simulink model "FPIDUpravlenie"  (Simulink 7.7)
settings: Solver=ode23t  StartTime=0.0  StopTime=50  RelTol=1e-3
values from neighbouring files (symbols this model uses):
  control_a = [-1,-0.975000000000000,-0.950000000000000,-0.925000000000000,-0.900000000000000,-0.875000000000000,-0.850000000000000,-0.825000000000000,-0.800000000000000,-0.775000000000000,-0.750000000000000,-0.725000000000000,-0.700000000000000,-0.675000000000000,-0.650000000000000,-0.625000000000000,-0.600000000000000,-0.575000000000000,-0.550000000000000,-0.525000000000000,-0.500000000000000,-0.4750000000000 ...(+1058 chars)    [main.m]
  control_p = [-1,-0.975000000000000,-0.950000000000000,-0.925000000000000,-0.900000000000000,-0.875000000000000,-0.850000000000000,-0.825000000000000,-0.800000000000000,-0.775000000000000,-0.750000000000000,-0.725000000000000,-0.700000000000000,-0.675000000000000,-0.650000000000000,-0.625000000000000,-0.600000000000000,-0.575000000000000,-0.550000000000000,-0.525000000000000,-0.500000000000000,-0.4750000000000 ...(+1058 chars)    [main.m]
  force_a = [-1.11662323915155,-1.09378407342940,-1.07265330175950,-1.04325193963191,-1.01132720072323,-0.977223749190414,-0.938313974120250,-0.915271484375000,-0.878089162348878,-0.843089432210708,-0.808883264518567,-0.764209831066494,-0.722158864286485,-0.679419665506261,-0.643924317249568,-0.610622608349525,-0.566994046173359,-0.526776706201425,-0.495851299384715,-0.457681114394430,-0.413805712974957,-0.38 ...(+1125 chars)    [main.m]
  force_p = [-0.714170782059585,-0.698541481136658,-0.676359428972366,-0.657306593399180,-0.636149510200777,-0.615949677515112,-0.602138570676813,-0.585879142379102,-0.565408182885363,-0.543655801354706,-0.527755120628238,-0.502405059234672,-0.485276085519214,-0.468134124703152,-0.445933772533463,-0.427151136118307,-0.408462867012090,-0.386931266191710,-0.367853637062824,-0.349068470693005,-0.324248856460492, ...(+1121 chars)    [main.m]
  Kpa = 0.7*Kua    (= 0.465009225034)    [main.m]
  Kpp = 0.33*Kup    (= 0.127856690685)    [main.m]
  rpm_a = [-7339.45782001209,-7212.46690016528,-7085.45931302586,-6928.76328688402,-6788.57281024633,-6657.59465144230,-6511.41380896936,-6365.92031625604,-6207.93597881609,-6041.64663461541,-5911.49080716649,-5761.94058931792,-5622.99053485574,-5477.24984975964,-5308.98813100961,-5148.14194899341,-4993.59811636119,-4838.25096717246,-4657.71766075724,-4490.92806302583,-4332.56953312800,-4153.59004094051,-39 ...(+1020 chars)    [main.m]
  rpm_p = [-3941.33990805745,-3812.34781047405,-3751.11151919774,-3716.53325007516,-3652.15015900441,-3605.21060614596,-3541.61821912219,-3501.87845652477,-3434.16395565290,-3361.65746230900,-3323.64747018525,-3262.37352633531,-3200.40694372361,-3113.97714681560,-3066.79116629220,-2985.72573717380,-2938.26747796475,-2854.00073711688,-2797.89727840112,-2739.44446768238,-2641.03778047718,-2564.22034843818,-24 ...(+1020 chars)    [main.m]
  Tda = 0.15*Tua    (= 1.125)    [main.m]
  Tdp = 0.33*Tup    (= 0.825)    [main.m]
  Tia = 0.4*Tua    (= 3)    [main.m]
  Tip = 0.5*Tup    (= 1.25)    [main.m]
  Ts = 0.1    [main.m]
undefined symbols (not defined in the file or in its folder): DiscIntNeverNeededParam
libraries: simulink x6, fuzblock x2
settings Model: Creator=melanholly  LastModifiedBy=melanholly
settings SolverCC: ShapePreserveControl=EnableAll  SolverResetMethod=Robust

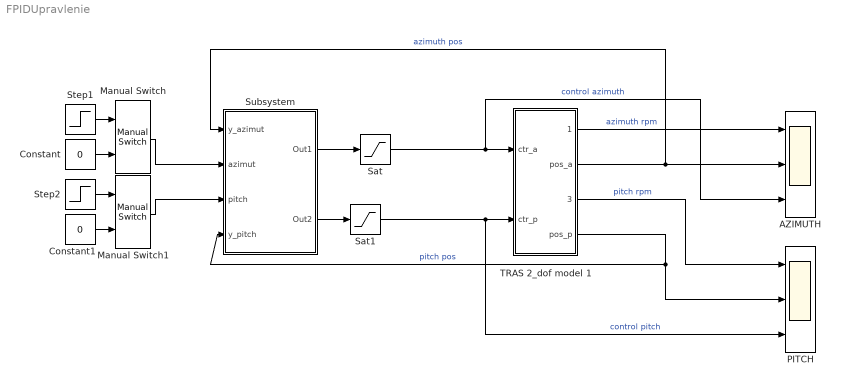
== system FPIDUpravlenie ==
  AZIMUTH : Scope  NumInputPorts=3
      settings: TimeRange=50  YMin=-3000~0~-0.4  YMax=3000~1.5~0.4
  Constant : Constant  Value=0
  Constant1 : Constant  Value=0
  Manual Switch : simulink/Signal Routing/Manual Switch  SystemSampleTime=-1  sw=1  action=0  varsize=off
  Manual Switch1 : simulink/Signal Routing/Manual Switch  SystemSampleTime=-1  sw=1  action=0  varsize=off
  PITCH : Scope  NumInputPorts=3
      settings: TimeRange=50  YMin=0~-2~0.2  YMax=4000~2~1
  Sat : Saturate  UpperLimit=0.3  LowerLimit=-0.3
  Sat1 : Saturate  UpperLimit=1  LowerLimit=.2
  Step1 : Step  After=0.3  SampleTime=0
  Step2 : Step  After=0.3  SampleTime=0
  Subsystem : Subsystem  mask{Kp_a=Kpa, Ki_a=Kpa/Tia, Kd_a=Kpa*Tda, Kp2=0, Ti2=0, Td2=0.2, N2=1, Kp3=0, Ti3=0, Td3=0.2, N3=1, Kp_p=Kpp, Ki_p=Kpp/Tip, Kd_p=Kpp*Tdp}
      mask prompts: Kp_a "Kp"; Ki_a "Ki"; Kd_a "Kd"; Kp2 "Kp"; Ti2 "Ti"; Td2 "Td"; N2 "N"; Kp3 "Kp"; Ti3 "Ti"; Td3 "Td"; N3 "N"; Kp_p "Kp"; Ki_p "Ki"; Kd_p "Kd"
      mask init:
      | GE_a = 1;
      | GCE_a = GE_a*(Kp_a-sqrt(Kp_a^2-4*Ki_a*Kd_a))/2/Ki_a;
      | GCU_a = Ki_a/GE_a;
      | GU_a = Kd_a/GCE_a;
      | if imag(GCE_a)~=0
      | error('GCE_a e kompleksno chislo molq promenenete koeficientite za nego');
      | end
      | 
      | GE_p = 1;
      | GCE_p = GE_p*(Kp_p-sqrt(Kp_p^2-4*Ki_p*Kd_p))/2/Ki_p;
      | GCU_p = Ki_p/GE_p;
      | GU_p = Kd_p/GCE_p;
      | 
      | if imag(GCE_p)~=0
      | error('GCE_p e kompleksno chislo molq promenenete koeficientite za nego');
      | end
      mask TabNameString: Azimut,Azimut,Azimut,hv,hv,hv,hv,vh,vh,vh,vh,Pitch,Pitch,Pitch
      mask Display:
      | disp Control
      | port_label('input', 1, 'a_y');
      | port_label('input', 2, 'a_r');
      | port_label('input', 3, 'p_r');
      | port_label('input', 4, 'p_y');
      | port_label('output', 1, 'ac');
      | port_label('output', 2, 'pc');
  TRAS 2_dof model 1 : Subsystem
  wires:
  TRAS 2_dof model 1/1(rpm_a) -> AZIMUTH/1  "azimuth rpm"
  TRAS 2_dof model 1/2(pos_a) -> AZIMUTH/2, Subsystem/1(y_azimut)  "azimuth pos"
  Step1/1 -> Manual Switch/1
  Constant/1 -> Manual Switch/2
  Step2/1 -> Manual Switch1/1
  Constant1/1 -> Manual Switch1/2
  TRAS 2_dof model 1/3(rpm_p) -> PITCH/1  "pitch rpm"
  TRAS 2_dof model 1/4(pos_p) -> PITCH/2, Subsystem/4(y_pitch)  "pitch pos"
  Manual Switch1/1 -> Subsystem/3(pitch)
  Subsystem/1(Out1) -> Sat/1
  Manual Switch/1 -> Subsystem/2(azimut)
  Sat1/1 -> PITCH/3, TRAS 2_dof model 1/2(ctr_p)  "control pitch"
  Sat/1 -> AZIMUTH/3, TRAS 2_dof model 1/1(ctr_a)  "control azimuth"
  Subsystem/2(Out2) -> Sat1/1

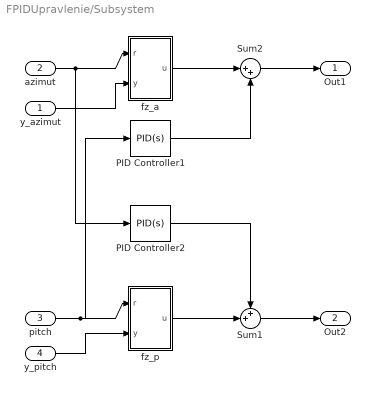
== system FPIDUpravlenie/Subsystem ==
  y_azimut : Inport
  azimut : Inport  Port=2
  pitch : Inport  Port=3
  y_pitch : Inport  Port=4
  PID Controller1 : simulink/Continuous/PID Controller  SystemSampleTime=-1  Controller=PID  TimeDomain=Continuous-time  SampleTime=1  IntegratorMethod=Forward Euler  FilterMethod=Forward Euler  Form=Ideal  P=Kp2  I=Ti2  D=Td2  N=N2  InitialConditionSource=internal  InitialConditionForIntegrator=0  InitialConditionForFilter=0  ExternalReset=none  LimitOutput=off  UpperSaturationLimit=inf  LowerSaturationLimit=-inf  LinearizeAsGain=off  AntiWindupMode=none  Kb=1  TrackingMode=off  Kt=1  PParamMin=[]  PParamMax=[]  IParamMin=[]  IParamMax=[]  DParamMin=[]  DParamMax=[]  NParamMin=[]  NParamMax=[]  KbParamMin=[]  KbParamMax=[]  KtParamMin=[]  KtParamMax=[]  POutMin=[]  POutMax=[]  IOutMin=[]  IOutMax=[]  DOutMin=[]  DOutMax=[]  NOutMin=[]  NOutMax=[]  KbOutMin=[]  KbOutMax=[]  KtOutMin=[]  KtOutMax=[]  IntegratorOutMin=[]  IntegratorOutMax=[]  FilterOutMin=[]  FilterOutMax=[]  SumOutMin=[]  SumOutMax=[]  SumI1OutMin=[]  SumI1OutMax=[]  SumI2OutMin=[]  SumI2OutMax=[]  SumI3OutMin=[]  SumI3OutMax=[]  SumDOutMin=[]  SumDOutMax=[]  SaturationOutMin=[]  SaturationOutMax=[]  IntegratorContinuousStateAttributes=''  IntegratorStateMustResolveToSignalObject=off  IntegratorRTWStateStorageClass=Auto  FilterContinuousStateAttributes=''  FilterStateMustResolveToSignalObject=off  FilterRTWStateStorageClass=Auto
  PID Controller2 : simulink/Continuous/PID Controller  SystemSampleTime=-1  Controller=PID  TimeDomain=Continuous-time  SampleTime=1  IntegratorMethod=Forward Euler  FilterMethod=Forward Euler  Form=Ideal  P=Kp3  I=Ti3  D=Td3  N=N3  InitialConditionSource=internal  InitialConditionForIntegrator=0  InitialConditionForFilter=0  ExternalReset=none  LimitOutput=off  UpperSaturationLimit=inf  LowerSaturationLimit=-inf  LinearizeAsGain=off  AntiWindupMode=none  Kb=1  TrackingMode=off  Kt=1  PParamMin=[]  PParamMax=[]  IParamMin=[]  IParamMax=[]  DParamMin=[]  DParamMax=[]  NParamMin=[]  NParamMax=[]  KbParamMin=[]  KbParamMax=[]  KtParamMin=[]  KtParamMax=[]  POutMin=[]  POutMax=[]  IOutMin=[]  IOutMax=[]  DOutMin=[]  DOutMax=[]  NOutMin=[]  NOutMax=[]  KbOutMin=[]  KbOutMax=[]  KtOutMin=[]  KtOutMax=[]  IntegratorOutMin=[]  IntegratorOutMax=[]  FilterOutMin=[]  FilterOutMax=[]  SumOutMin=[]  SumOutMax=[]  SumI1OutMin=[]  SumI1OutMax=[]  SumI2OutMin=[]  SumI2OutMax=[]  SumI3OutMin=[]  SumI3OutMax=[]  SumDOutMin=[]  SumDOutMax=[]  SaturationOutMin=[]  SaturationOutMax=[]  IntegratorContinuousStateAttributes=''  IntegratorStateMustResolveToSignalObject=off  IntegratorRTWStateStorageClass=Auto  FilterContinuousStateAttributes=''  FilterStateMustResolveToSignalObject=off  FilterRTWStateStorageClass=Auto
  Sum1 : Sum  Inputs=++|
  Sum2 : Sum  Inputs=|++
  fz_a : Subsystem
  fz_p : Subsystem
  Out1 : Outport
  Out2 : Outport  Port=2
  wires:
  azimut/1 -> PID Controller2/1, fz_a/1(r)
  pitch/1 -> PID Controller1/1, fz_p/1(r)
  PID Controller2/1 -> Sum1/1
  fz_p/1(u) -> Sum1/2
  Sum1/1 -> Out2/1
  fz_a/1(u) -> Sum2/1
  Sum2/1 -> Out1/1
  PID Controller1/1 -> Sum2/2
  y_azimut/1 -> fz_a/2(y)
  y_pitch/1 -> fz_p/2(y)

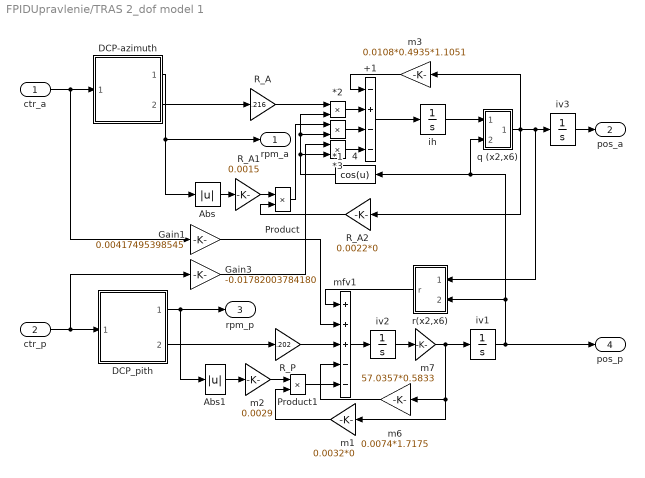
== system FPIDUpravlenie/TRAS 2_dof model 1 ==
  ctr_a : Inport
  ctr_p : Inport  Port=2
  *1 : Product  SaturateOnIntegerOverflow=on  InputSameDT=on  OutDataTypeStr=Inherit: Same as first input
  *2 : Product  SaturateOnIntegerOverflow=on  InputSameDT=on  OutDataTypeStr=Inherit: Same as first input
  *3 : Product  SaturateOnIntegerOverflow=on  InputSameDT=on  OutDataTypeStr=Inherit: Same as first input
  +1 : Sum  Inputs=-+--  SaturateOnIntegerOverflow=on  InputSameDT=on  OutDataTypeStr=Inherit: Same as first input
  4 : Fcn  Expr=cos(u)
  Abs : Abs  SaturateOnIntegerOverflow=on
  Abs1 : Abs  SaturateOnIntegerOverflow=on
  DCP-azimuth : Subsystem
  DCP_pith : Subsystem
  Gain1 : Gain  Gain=0.00417495398545  SaturateOnIntegerOverflow=on  OutDataTypeStr=Inherit: Same as input  ParamDataTypeStr=Inherit: Same as input
  Gain3 : Gain  Gain=-0.01782003784180  SaturateOnIntegerOverflow=on  OutDataTypeStr=Inherit: Same as input  ParamDataTypeStr=Inherit: Same as input
  Product : Product  SaturateOnIntegerOverflow=on  InputSameDT=on  OutDataTypeStr=Inherit: Same as first input
  Product1 : Product  SaturateOnIntegerOverflow=on  OutDataTypeStr=Inherit: Same as first input
  R_A : Gain  Gain=.216  OutDataTypeStr=Inherit: Same as input  ParamDataTypeStr=Inherit: Same as input
  R_A1 : Gain  Gain=0.0015  OutDataTypeStr=Inherit: Same as input  ParamDataTypeStr=Inherit: Same as input
  R_A2 : Gain  Gain=0.0022*0  OutDataTypeStr=Inherit: Same as input  ParamDataTypeStr=Inherit: Same as input
  R_P : Gain  Gain=.202  OutDataTypeStr=Inherit: Same as input  ParamDataTypeStr=Inherit: Same as input
  ih : Integrator  UpperSaturationLimit=10  LowerSaturationLimit=-10
  iv1 : Integrator  LimitOutput=on  UpperSaturationLimit=pi/2  LowerSaturationLimit=-pi/2
  iv2 : Integrator  UpperSaturationLimit=pi  LowerSaturationLimit=-pi
  iv3 : Integrator  LimitOutput=on  UpperSaturationLimit=6  LowerSaturationLimit=-6
  m1 : Gain  Gain=0.0032*0  SaturateOnIntegerOverflow=on  OutDataTypeStr=Inherit: Same as input  ParamDataTypeStr=Inherit: Same as input
  m2 : Gain  Gain=0.0029  SaturateOnIntegerOverflow=on  OutDataTypeStr=Inherit: Same as input  ParamDataTypeStr=Inherit: Same as input
  m3 : Gain  Gain=0.0108*0.4935*1.1051  OutDataTypeStr=Inherit: Same as input  ParamDataTypeStr=Inherit: Same as input
  m6 : Gain  Gain=0.0074*1.7175  OutDataTypeStr=Inherit: Same as input  ParamDataTypeStr=Inherit: Same as input
  m7 : Gain  Gain=57.0357*0.5833  SaturateOnIntegerOverflow=on  OutDataTypeStr=Inherit: Same as input  ParamDataTypeStr=Inherit: Same as input
  mfv1 : Sum  Inputs=+++--  SaturateOnIntegerOverflow=on  InputSameDT=on  OutDataTypeStr=Inherit: Same as first input
  q (x2,x6) : Subsystem
  r(x2,x6) : Subsystem
  rpm_a : Outport
  pos_a : Outport  Port=2
  rpm_p : Outport  Port=3
  pos_p : Outport  Port=4
  wires:
  DCP-azimuth/1(RPM_A) -> Abs/1, rpm_a/1
  +1/1 -> ih/1
  iv3/1 -> pos_a/1
  ctr_p/1 -> Gain3/1, DCP_pith/1(CTR_P)
  ctr_a/1 -> Gain1/1, DCP-azimuth/1(CTR_A)
  Gain3/1 -> *3/1
  Gain1/1 -> mfv1/2
  4/1 -> *3/2, *1/2, *2/2
  Product/1 -> *1/1
  *3/1 -> +1/4
  m2/1 -> Product1/1
  m1/1 -> Product1/2
  iv1/1 -> q (x2,x6)/2(x6), 4/1, r(x2,x6)/2(x6), pos_p/1
  R_P/1 -> mfv1/3
  r(x2,x6)/1(r) -> mfv1/1
  Product1/1 -> mfv1/5
  Abs1/1 -> m2/1
  DCP_pith/1(RPM_P) -> rpm_p/1, Abs1/1
  m7/1 -> m1/1, m6/1, iv1/1
  mfv1/1 -> iv2/1
  iv2/1 -> m7/1
  m6/1 -> mfv1/4
  DCP_pith/2(FORCE_P) -> R_P/1
  R_A2/1 -> Product/2
  R_A1/1 -> Product/1
  Abs/1 -> R_A1/1
  R_A/1 -> *2/1
  q (x2,x6)/1(q) -> R_A2/1, m3/1, r(x2,x6)/1(y2), iv3/1
  ih/1 -> q (x2,x6)/1(x2)
  *2/1 -> +1/2
  m3/1 -> +1/1
  *1/1 -> +1/3
  DCP-azimuth/2(FORCE_A) -> R_A/1

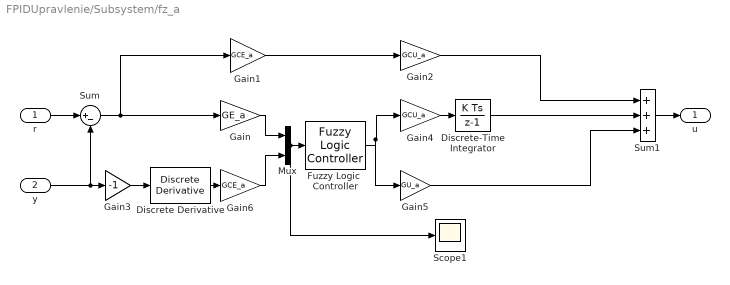
== system FPIDUpravlenie/Subsystem/fz_a ==
  r : Inport
  y : Inport  Port=2
  Discrete Derivative : simulink/Discrete/Discrete Derivative  SystemSampleTime=-1  gainval=1.0  ICPrevScaledInput=0.0  OutMin=[]  OutMax=[]  OutDataType=fixdt(1, 16)  OutScaling=2^-10  DoSatur=off
  Discrete-Time Integrator : DiscreteIntegrator  SampleTime=Ts  ICPrevOutput=DiscIntNeverNeededParam  ICPrevScaledInput=DiscIntNeverNeededParam
  Fuzzy Logic  Controller : fuzblock/Fuzzy Logic  Controller  SystemSampleTime=-1  fis=FIS
  Gain : Gain  Gain=GE_a  SampleTime=Ts
  Gain1 : Gain  Gain=GCE_a  SampleTime=Ts
  Gain2 : Gain  Gain=GCU_a  SampleTime=Ts
  Gain3 : Gain  Gain=-1  SampleTime=Ts
  Gain4 : Gain  Gain=GCU_a  SampleTime=Ts
  Gain5 : Gain  Gain=GU_a  SampleTime=Ts
  Gain6 : Gain  Gain=GCE_a  SampleTime=Ts
  Mux : Mux  Inputs=2
  Scope1 : Scope
      settings: TimeRange=12  YMin=0  YMax=1.223758865248227  SaveName=ScopeData2
  Sum : Sum  Inputs=|+-
  Sum1 : Sum  Inputs=+++
  u : Outport
  wires:
  Sum1/1 -> u/1
  r/1 -> Sum/1
  Gain3/1 -> Discrete Derivative/1
  Fuzzy Logic  Controller/1 -> Gain5/1, Gain4/1
  Discrete-Time Integrator/1 -> Sum1/2
  Sum/1 -> Gain/1, Gain1/1
  y/1 -> Gain3/1, Sum/2
  Gain1/1 -> Gain2/1
  Gain2/1 -> Sum1/1
  Gain4/1 -> Discrete-Time Integrator/1
  Gain5/1 -> Sum1/3
  Discrete Derivative/1 -> Gain6/1
  Mux/1 -> Scope1/1, Fuzzy Logic  Controller/1
  Gain/1 -> Mux/1
  Gain6/1 -> Mux/2

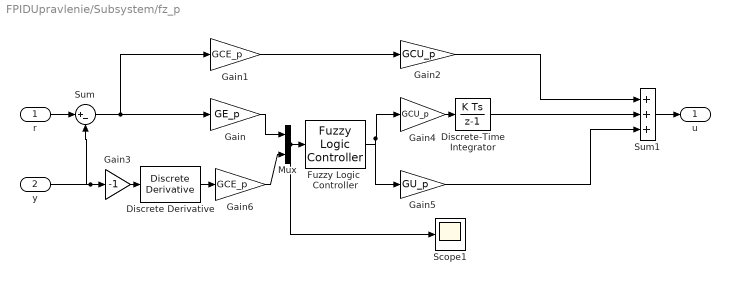
== system FPIDUpravlenie/Subsystem/fz_p ==
  r : Inport
  y : Inport  Port=2
  Discrete Derivative : simulink/Discrete/Discrete Derivative  SystemSampleTime=-1  gainval=1.0  ICPrevScaledInput=0.0  OutMin=[]  OutMax=[]  OutDataType=fixdt(1, 16)  OutScaling=2^-10  DoSatur=off
  Discrete-Time Integrator : DiscreteIntegrator  SampleTime=Ts  ICPrevOutput=DiscIntNeverNeededParam  ICPrevScaledInput=DiscIntNeverNeededParam
  Fuzzy Logic  Controller : fuzblock/Fuzzy Logic  Controller  SystemSampleTime=-1  fis=FIS
  Gain : Gain  Gain=GE_p  SampleTime=Ts
  Gain1 : Gain  Gain=GCE_p  SampleTime=Ts
  Gain2 : Gain  Gain=GCU_p  SampleTime=Ts
  Gain3 : Gain  Gain=-1  SampleTime=Ts
  Gain4 : Gain  Gain=GCU_p  SampleTime=Ts
  Gain5 : Gain  Gain=GU_p  SampleTime=Ts
  Gain6 : Gain  Gain=GCE_p  SampleTime=Ts
  Mux : Mux  Inputs=2
  Scope1 : Scope
      settings: TimeRange=12  YMin=0  YMax=1.223758865248227  SaveName=ScopeData2
  Sum : Sum  Inputs=|+-
  Sum1 : Sum  Inputs=+++
  u : Outport
  wires:
  Sum1/1 -> u/1
  r/1 -> Sum/1
  Gain3/1 -> Discrete Derivative/1
  Fuzzy Logic  Controller/1 -> Gain5/1, Gain4/1
  Discrete-Time Integrator/1 -> Sum1/2
  Sum/1 -> Gain/1, Gain1/1
  y/1 -> Gain3/1, Sum/2
  Gain1/1 -> Gain2/1
  Gain2/1 -> Sum1/1
  Gain4/1 -> Discrete-Time Integrator/1
  Gain5/1 -> Sum1/3
  Discrete Derivative/1 -> Gain6/1
  Mux/1 -> Scope1/1, Fuzzy Logic  Controller/1
  Gain/1 -> Mux/1
  Gain6/1 -> Mux/2

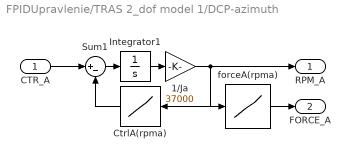
== system FPIDUpravlenie/TRAS 2_dof model 1/DCP-azimuth ==
  CTR_A : Inport
  1/Ja : Gain  Gain=37000  SaturateOnIntegerOverflow=on  OutDataTypeStr=Inherit: Same as input  ParamDataTypeStr=Inherit: Same as input
  CtrlA(rpma) : Lookup  InputValues=rpm_a  Table=control_a  SaturateOnIntegerOverflow=on
  Integrator1 : Integrator
  Sum1 : Sum  Inputs=|+-  SaturateOnIntegerOverflow=on  InputSameDT=on  OutDataTypeStr=Inherit: Same as first input
  forceA(rpma) : Lookup  InputValues=rpm_a  Table=force_a  SaturateOnIntegerOverflow=on
  RPM_A : Outport
  FORCE_A : Outport  Port=2
  wires:
  forceA(rpma)/1 -> FORCE_A/1
  CTR_A/1 -> Sum1/1
  1/Ja/1 -> RPM_A/1, forceA(rpma)/1, CtrlA(rpma)/1
  Integrator1/1 -> 1/Ja/1
  CtrlA(rpma)/1 -> Sum1/2
  Sum1/1 -> Integrator1/1

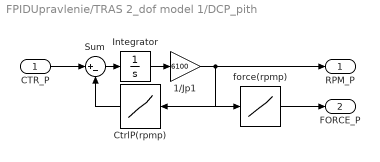
== system FPIDUpravlenie/TRAS 2_dof model 1/DCP_pith ==
  CTR_P : Inport
  1/Jp1 : Gain  Gain=6100  OutDataTypeStr=Inherit: Same as input  ParamDataTypeStr=Inherit: Same as input
  CtrlP(rpmp) : Lookup  InputValues=rpm_p  Table=control_p  SaturateOnIntegerOverflow=on
  Integrator : Integrator
  Sum : Sum  Inputs=|+-  SaturateOnIntegerOverflow=on  InputSameDT=on  OutDataTypeStr=Inherit: Same as first input
  force(rpmp) : Lookup  InputValues=rpm_p  Table=force_p  SaturateOnIntegerOverflow=on
  RPM_P : Outport
  FORCE_P : Outport  Port=2
  wires:
  force(rpmp)/1 -> FORCE_P/1
  CTR_P/1 -> Sum/1
  1/Jp1/1 -> RPM_P/1, force(rpmp)/1, CtrlP(rpmp)/1
  CtrlP(rpmp)/1 -> Sum/2
  Integrator/1 -> 1/Jp1/1
  Sum/1 -> Integrator/1

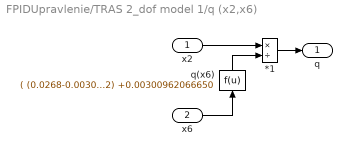
== system FPIDUpravlenie/TRAS 2_dof model 1/q (x2,x6) ==
  x2 : Inport
  x6 : Inport  Port=2
  " q(x6)" : Fcn  Expr=( (0.0268-0.00300962066650)*cos(u)^2) +0.00300962066650
  *1 : Product  Inputs=*/  SaturateOnIntegerOverflow=on  InputSameDT=on  OutDataTypeStr=Inherit: Same as first input
  q : Outport
  wires:
  " q(x6)"/1 -> *1/2
  x6/1 -> " q(x6)"/1
  x2/1 -> *1/1
  *1/1 -> q/1

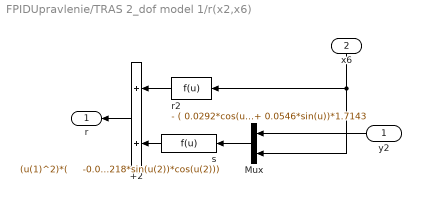
== system FPIDUpravlenie/TRAS 2_dof model 1/r(x2,x6) ==
  y2 : Inport
  x6 : Inport  Port=2
  +2 : Sum  SaturateOnIntegerOverflow=on  InputSameDT=on  OutDataTypeStr=Inherit: Same as first input
  Mux : Mux  Inputs=2
  r2 : Fcn  Expr=- ( 0.0292*cos(u)+ 0.0546*sin(u))*1.7143
  s : Fcn  Expr="(u(1)^2)*(     -0.07389953104162*  0.28753198180218*sin(u(2))*cos(u(2)))"
  r : Outport
  wires:
  y2/1 -> Mux/1
  +2/1 -> r/1
  x6/1 -> r2/1, Mux/2
  s/1 -> +2/2
  r2/1 -> +2/1
  Mux/1 -> s/1
